simulink model "cluster7"  (R2016a)
settings: Solver=FixedStepAuto  StartTime=0.0  StopTime=10  FixedStep=0.001  RelTol=1e-3
InitFcn:
  | clear;
  | clc;
  | R = 1/2;
  | L = 1;
  | L1 = [-1 0 1;1 -1 0;0 1 -1];
  | 
  | gammar = 0.75;
  | L1 = [L1,gammar*L1];
  | Xx = [0 10 5]';
  | Vx = [0.5 0.2 0.3]';
  | Xy = [2 2 10]';
  | Vy = [0.1 0.3 0.4];
  | Vxend = [0 0 0]';
  | Vyend = [0 0 0]';
  | Xend = [3 4 5]';
  | Yend = [3 4 5]';
StopFcn:
  | plot(X1_1(:,2),X1_1(:,5),X1_1(:,3),X1_1(:,6),X1_1(:,4),X1_1(:,7));
  | hold on
  | grid on
  | xlabel('x')
  | ylabel('y')
  | N = size(X1_1,1);
  | for i=1:N/40;
  |     cla;
  |     k = 40*i;
  |     plot(X1_1(:,2),X1_1(:,5),X1_1(:,3),X1_1(:,6),X1_1(:,4),X1_1(:,7));
  |     plot(X1_1(k,2),X1_1(k,5),'o',X1_1(k,3),X1_1(k,6),'o',X1_1(k,4),X1_1(k,7),'o');
  |     frame=getframe(gcf);
  |     imind=frame2im(frame);
  | 
  | end
settings Model: Creator=Administrator  LastModifiedBy=Administrator

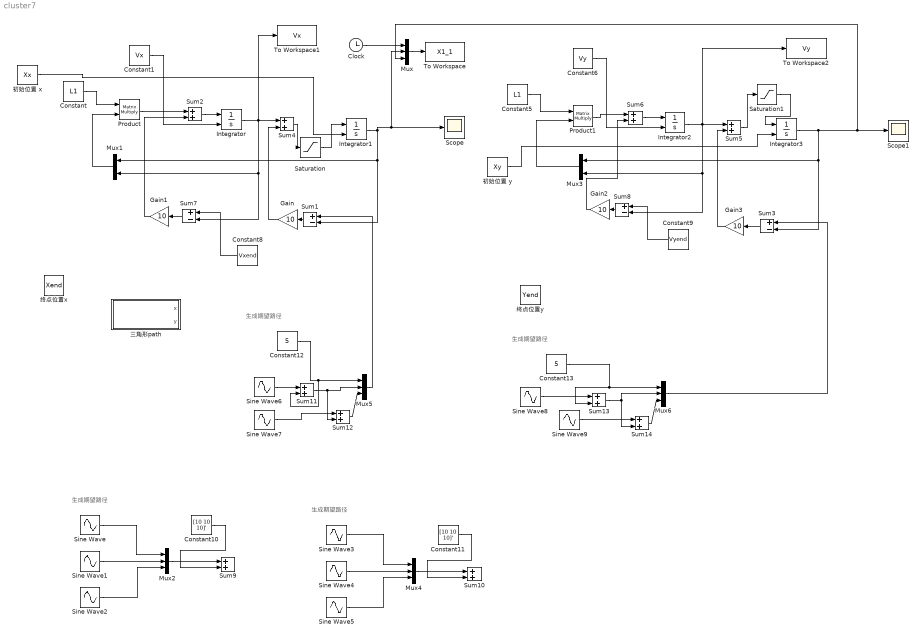
== system cluster7 ==
  note: 生成期望路径
  note: 生成期望路径
  note: 生成期望路径
  note: 生成期望路径
  Clock : Clock
      settings: Decimation=100
  Constant : Constant  Value=L1  VectorParams1D=off
  Constant1 : Constant  Value=Vx
  Constant10 : Constant  Value=[10 10 10]'
  Constant11 : Constant  Value=[10 10 10]'
  Constant12 : Constant  Value=5
  Constant13 : Constant  Value=5
  Constant5 : Constant  Value=L1  VectorParams1D=off
  Constant6 : Constant  Value=Vy
  Constant8 : Constant  Value=Vxend
  Constant9 : Constant  Value=Vyend
  Gain{,1..3} (4 alike) : Gain  Gain=10
  Integrator{,1..3} (4 alike) : Integrator  InitialConditionSource=external
  Mux{,2,4..6} (5 alike) : Mux  Inputs=3
  Mux1 : Mux  Inputs=2
  Mux3 : Mux  Inputs=2
  Product : Product  Multiplication=Matrix(*)
  Product1 : Product  Multiplication=Matrix(*)
  Saturation : Saturate  UpperLimit=5  LowerLimit=-5
  Saturation1 : Saturate  UpperLimit=5  LowerLimit=-5
  Scope : Scope
  Scope1 : Scope
  Sine Wave : Sin  Amplitude=2  SampleTime=0
  Sine Wave1 : Sin  Amplitude=2  Phase=120*pi/180  SampleTime=0
  Sine Wave2 : Sin  Amplitude=2  Phase=240*pi/180  SampleTime=0
  Sine Wave3 : Sin  Amplitude=2  Phase=90*pi/180  SampleTime=0
  Sine Wave4 : Sin  Amplitude=2  Phase=210*pi/180  SampleTime=0
  Sine Wave5 : Sin  Amplitude=2  Phase=330*pi/180  SampleTime=0
  Sine Wave6 : Sin  Amplitude=2  SampleTime=0
  Sine Wave7 : Sin  Amplitude=0.5  Frequency=20  SampleTime=0
  Sine Wave8 : Sin  Amplitude=2  Phase=90*pi/180  SampleTime=0
  Sine Wave9 : Sin  Amplitude=0.5  Frequency=20  Phase=90*pi/180  SampleTime=0
  Sum{1,3,7..8} (4 alike) : Sum  Inputs=+-
  Sum{2,4..6,9..14} (10 alike) : Sum
  To Workspace : ToWorkspace  VariableName=X1_1  SampleTime=-1
  To Workspace1 : ToWorkspace  VariableName=Vx  SampleTime=-1
  To Workspace2 : ToWorkspace  VariableName=Vy  SampleTime=-1
  三角形path : Subsystem
  初始位置 x : Constant  Value=Xx
  初始位置 y : Constant  Value=Xy
  终点位置x : Constant  Value=Xend
  终点位置y : Constant  Value=Yend
  wires:
  Constant/1 -> Product/1
  Constant1/1 -> Integrator/2
  Clock/1 -> Mux/1
  Mux/1 -> To Workspace/1
  初始位置 x/1 -> Integrator1/2
  Integrator1/1 -> Mux/2, Scope/1, Sum1/2, Mux1/1
  Mux1/1 -> Product/2
  Product/1 -> Sum2/1
  Sum2/1 -> Integrator/1
  Constant5/1 -> Product1/1
  Constant6/1 -> Integrator2/2
  初始位置 y/1 -> Integrator3/2
  Integrator3/1 -> Sum3/2, Mux3/1, Mux/3, Scope1/1
  Mux3/1 -> Product1/2
  Product1/1 -> Sum6/1
  Sum6/1 -> Integrator2/1
  Sum4/1 -> Saturation/1
  Sum5/1 -> Saturation1/1
  Integrator/1 -> To Workspace1/1, Sum4/1, Sum7/2, Mux1/2
  Constant8/1 -> Sum7/1
  Integrator2/1 -> To Workspace2/1, Sum8/2, Mux3/2, Sum5/1
  Constant9/1 -> Sum8/1
  Sum1/1 -> Gain/1
  Sum7/1 -> Gain1/1
  Sum8/1 -> Gain2/1
  Sum3/1 -> Gain3/1
  Gain/1 -> Sum4/2
  Gain3/1 -> Sum5/2
  Sine Wave/1 -> Mux2/1
  Sine Wave1/1 -> Mux2/2
  Sine Wave2/1 -> Mux2/3
  Mux2/1 -> Sum9/1
  Constant10/1 -> Sum9/2
  Sine Wave3/1 -> Mux4/1
  Sine Wave4/1 -> Mux4/2
  Sine Wave5/1 -> Mux4/3
  Mux4/1 -> Sum10/1
  Constant11/1 -> Sum10/2
  Constant12/1 -> Mux5/1, Sum11/2
  Sine Wave6/1 -> Sum11/1
  Sine Wave7/1 -> Sum12/1
  Sum12/1 -> Mux5/3
  Constant13/1 -> Mux6/1, Sum13/2
  Sine Wave8/1 -> Sum13/1
  Sum13/1 -> Mux6/2, Sum14/2
  Sine Wave9/1 -> Sum14/1
  Sum14/1 -> Mux6/3
  Gain1/1 -> Sum2/2
  Gain2/1 -> Sum6/2
  Sum11/1 -> Sum12/2, Mux5/2
  Mux5/1 -> Sum1/1
  Mux6/1 -> Sum3/1
  Saturation/1 -> Integrator1/1
  Saturation1/1 -> Integrator3/1

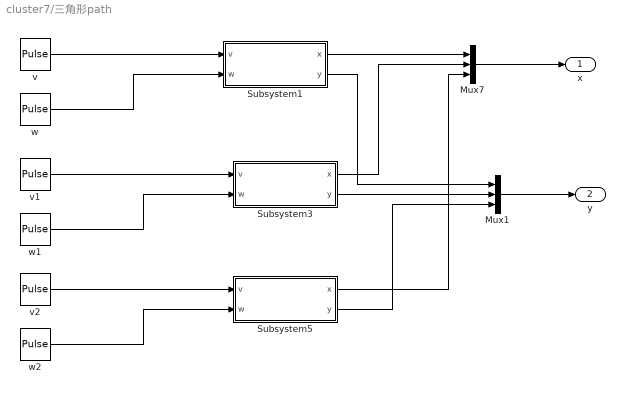
== system cluster7/三角形path ==
  Mux1 : Mux  Inputs=3
  Mux7 : Mux  Inputs=3
  Subsystem1 : Subsystem
  Subsystem3 : Subsystem
  Subsystem5 : Subsystem
  v : DiscretePulseGenerator  PulseType=Time based  Amplitude=5  PulseWidth=50
  v1 : DiscretePulseGenerator  PulseType=Time based  Amplitude=5  PulseWidth=50
  v2 : DiscretePulseGenerator  PulseType=Time based  Amplitude=5  PulseWidth=50
  w : DiscretePulseGenerator  PulseType=Time based  Amplitude=2*pi/3  PulseWidth=50  PhaseDelay=1
  w1 : DiscretePulseGenerator  PulseType=Time based  Amplitude=2*pi/3  PulseWidth=50  PhaseDelay=1
  w2 : DiscretePulseGenerator  PulseType=Time based  Amplitude=2*pi/3  PulseWidth=50  PhaseDelay=1
  x : Outport
  y : Outport  Port=2
  wires:
  Subsystem1/1(x) -> Mux7/1
  v/1 -> Subsystem1/1(v)
  w/1 -> Subsystem1/2(w)
  v1/1 -> Subsystem3/1(v)
  w1/1 -> Subsystem3/2(w)
  v2/1 -> Subsystem5/1(v)
  w2/1 -> Subsystem5/2(w)
  Subsystem3/1(x) -> Mux7/2
  Subsystem5/1(x) -> Mux7/3
  Subsystem1/2(y) -> Mux1/1
  Subsystem3/2(y) -> Mux1/2
  Subsystem5/2(y) -> Mux1/3
  Mux7/1 -> x/1
  Mux1/1 -> y/1

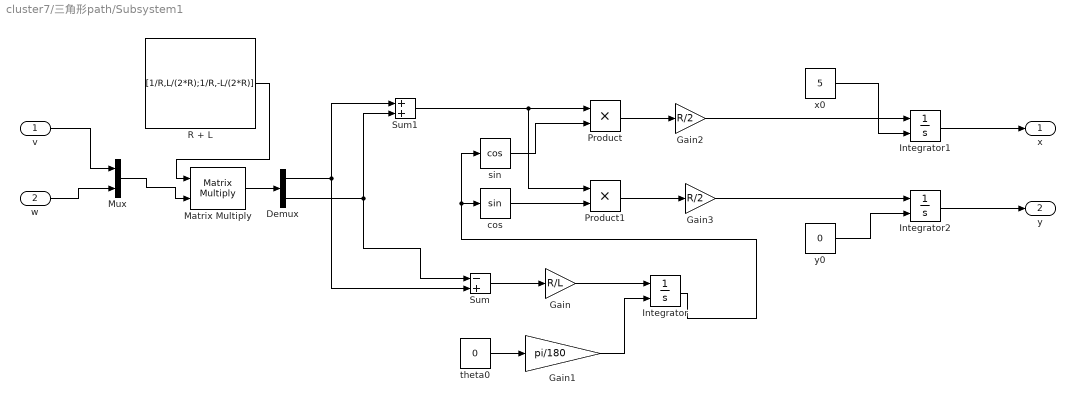
== system cluster7/三角形path/Subsystem1 ==
  v : Inport
  w : Inport  Port=2
  Demux : Demux  Outputs=2
  Gain : Gain  Gain=R/L
  Gain1 : Gain  Gain=pi/180
  Gain2 : Gain  Gain=R/2
  Gain3 : Gain  Gain=R/2
  Integrator : Integrator  InitialConditionSource=external
  Integrator1 : Integrator  InitialConditionSource=external
  Integrator2 : Integrator  InitialConditionSource=external
  Matrix Multiply : Product  Multiplication=Matrix(*)
  Mux : Mux  Inputs=2
  Product : Product
  Product1 : Product
  R + L : Constant  Value=[1/R,L/(2*R);1/R,-L/(2*R)]
  Sum : Sum  Inputs=-+
  Sum1 : Sum
  cos : Trigonometry
  sin : Trigonometry  Operator=cos
  theta0 : Constant  Value=0
  x0 : Constant  Value=5
  y0 : Constant  Value=0
  x : Outport
  y : Outport  Port=2
  wires:
  Demux/2 -> Sum/1, Sum1/2
  Demux/1 -> Sum1/1, Sum/2
  Sum/1 -> Gain/1
  Gain/1 -> Integrator/1
  Integrator/1 -> sin/1, cos/1
  theta0/1 -> Gain1/1
  Gain1/1 -> Integrator/2
  Sum1/1 -> Product1/1, Product/1
  sin/1 -> Product/2
  cos/1 -> Product1/2
  Product/1 -> Gain2/1
  Product1/1 -> Gain3/1
  Gain2/1 -> Integrator1/1
  Gain3/1 -> Integrator2/1
  y0/1 -> Integrator2/2
  x0/1 -> Integrator1/2
  Integrator1/1 -> x/1
  Integrator2/1 -> y/1
  v/1 -> Mux/1
  w/1 -> Mux/2
  Mux/1 -> Matrix Multiply/2
  Matrix Multiply/1 -> Demux/1
  R + L/1 -> Matrix Multiply/1

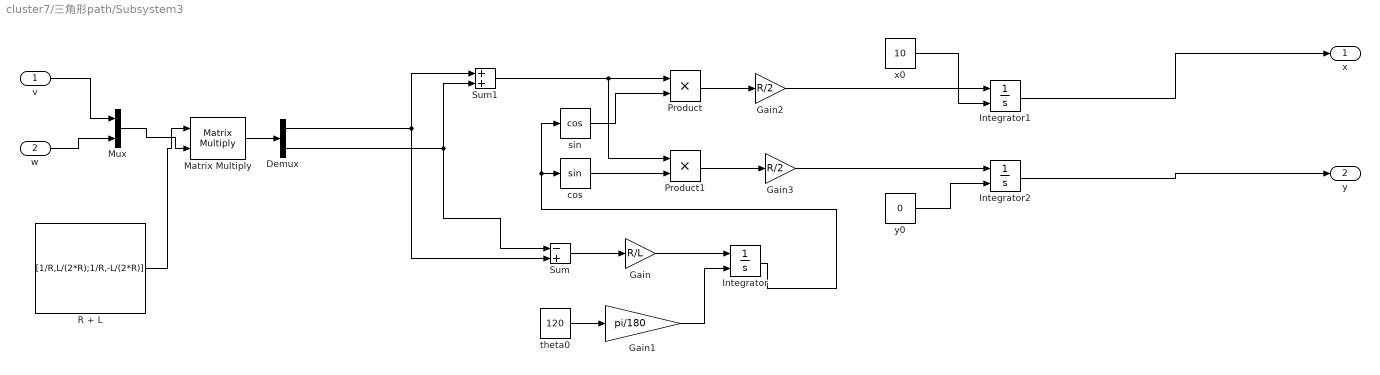
== system cluster7/三角形path/Subsystem3 ==
  v : Inport
  w : Inport  Port=2
  Demux : Demux  Outputs=2
  Gain : Gain  Gain=R/L
  Gain1 : Gain  Gain=pi/180
  Gain2 : Gain  Gain=R/2
  Gain3 : Gain  Gain=R/2
  Integrator : Integrator  InitialConditionSource=external
  Integrator1 : Integrator  InitialConditionSource=external
  Integrator2 : Integrator  InitialConditionSource=external
  Matrix Multiply : Product  Multiplication=Matrix(*)
  Mux : Mux  Inputs=2
  Product : Product
  Product1 : Product
  R + L : Constant  Value=[1/R,L/(2*R);1/R,-L/(2*R)]
  Sum : Sum  Inputs=-+
  Sum1 : Sum
  cos : Trigonometry
  sin : Trigonometry  Operator=cos
  theta0 : Constant  Value=120
  x0 : Constant  Value=10
  y0 : Constant  Value=0
  x : Outport
  y : Outport  Port=2
  wires:
  Demux/2 -> Sum/1, Sum1/2
  Demux/1 -> Sum1/1, Sum/2
  Sum/1 -> Gain/1
  Gain/1 -> Integrator/1
  Integrator/1 -> sin/1, cos/1
  theta0/1 -> Gain1/1
  Gain1/1 -> Integrator/2
  Sum1/1 -> Product1/1, Product/1
  sin/1 -> Product/2
  cos/1 -> Product1/2
  Product/1 -> Gain2/1
  Product1/1 -> Gain3/1
  Gain2/1 -> Integrator1/1
  Gain3/1 -> Integrator2/1
  y0/1 -> Integrator2/2
  x0/1 -> Integrator1/2
  Integrator1/1 -> x/1
  Integrator2/1 -> y/1
  v/1 -> Mux/1
  w/1 -> Mux/2
  Mux/1 -> Matrix Multiply/2
  Matrix Multiply/1 -> Demux/1
  R + L/1 -> Matrix Multiply/1

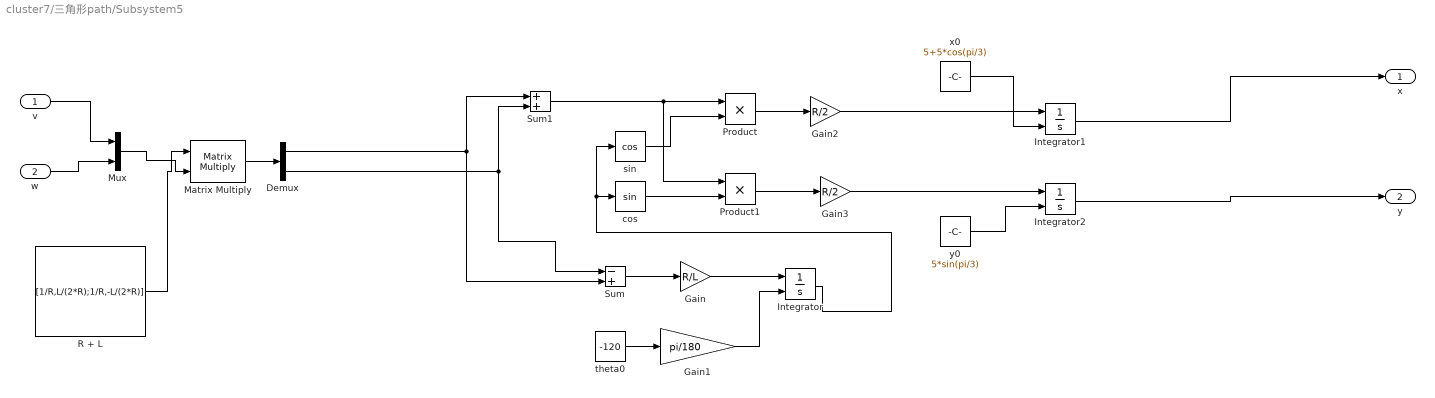
== system cluster7/三角形path/Subsystem5 ==
  v : Inport
  w : Inport  Port=2
  Demux : Demux  Outputs=2
  Gain : Gain  Gain=R/L
  Gain1 : Gain  Gain=pi/180
  Gain2 : Gain  Gain=R/2
  Gain3 : Gain  Gain=R/2
  Integrator : Integrator  InitialConditionSource=external
  Integrator1 : Integrator  InitialConditionSource=external
  Integrator2 : Integrator  InitialConditionSource=external
  Matrix Multiply : Product  Multiplication=Matrix(*)
  Mux : Mux  Inputs=2
  Product : Product
  Product1 : Product
  R + L : Constant  Value=[1/R,L/(2*R);1/R,-L/(2*R)]
  Sum : Sum  Inputs=-+
  Sum1 : Sum
  cos : Trigonometry
  sin : Trigonometry  Operator=cos
  theta0 : Constant  Value=-120
  x0 : Constant  Value=5+5*cos(pi/3)
  y0 : Constant  Value=5*sin(pi/3)
  x : Outport
  y : Outport  Port=2
  wires:
  Demux/2 -> Sum/1, Sum1/2
  Demux/1 -> Sum1/1, Sum/2
  Sum/1 -> Gain/1
  Gain/1 -> Integrator/1
  Integrator/1 -> sin/1, cos/1
  theta0/1 -> Gain1/1
  Gain1/1 -> Integrator/2
  Sum1/1 -> Product1/1, Product/1
  sin/1 -> Product/2
  cos/1 -> Product1/2
  Product/1 -> Gain2/1
  Product1/1 -> Gain3/1
  Gain2/1 -> Integrator1/1
  Gain3/1 -> Integrator2/1
  y0/1 -> Integrator2/2
  x0/1 -> Integrator1/2
  Integrator1/1 -> x/1
  Integrator2/1 -> y/1
  v/1 -> Mux/1
  w/1 -> Mux/2
  Mux/1 -> Matrix Multiply/2
  Matrix Multiply/1 -> Demux/1
  R + L/1 -> Matrix Multiply/1
